simulink model "AnalogOutput_model"  (R2016b)
settings: Solver=FixedStepAuto  StartTime=0.0  StopTime=tFinal  FixedStep=T  RelTol=1e-3  EnableMultiTasking=on
libraries: arduinolib x2
settings Model: SimulationMode=external  ExtModeTrigDuration=100  Creator=Christopher  LastModifiedBy=Christopher
settings DataIOCC: LimitDataPoints=on  StreamToWorkspace=on
settings OptimizationCC: LifeSpan=1  MaxStackSize=64
settings DebuggingCC: AllowSymbolicDim=off  SFUnexpectedBacktrackingDiag=warning  SFNoUnconditionalDefaultTransitionDiag=warning  SFExecutionAtInitializationDiag=none
settings HardwareCC: ProdBitPerPointer=32  ProdBitPerSizeT=32  ProdBitPerPtrDiffT=32  ProdLargestAtomicInteger=Long  ProdLargestAtomicFloat=Double  ProdWordSize=32  ProdHWDeviceType=ARM Compatible->ARM Cortex  UseEmbeddedCoderFeatures=off  UseSimulinkCoderFeatures=off
settings ModelReferenceCC: PropagateSignalLabelsOutOfModel=off
settings RTWCC: SystemTargetFile=ert.tlc  HardwareBoard=Arduino Due  TLCOptions=-aInlineSetEventsForThisBaseRateFcn=TLC_FALSE -aSuppressMultiTaskScheduler=TLC_FALSE -aRateBasedStepFcn=1  TemplateMakefile=ert_default_tmf  Description=Embedded Coder  RTWVerbose=off  Toolchain=Arduino ARM v1.6.7  BuildConfiguration=Faster Runs
settings CodeAppCC: MangleLength=10
settings ERTTargetCC: ERTCustomFileBanners=off  SupportContinuousTime=on  SupportNonInlinedSFcns=on  RemoveResetFunc=off  SupportVariableSizeSignals=on  ModelStepFunctionPrototypeControlCompliant=off  ExtMode=on  ExtModeMexArgs='127.0.0.1' 0 17725  ERTSrcFileBannerTemplate=codertarget_code_template.cgt  ERTHdrFileBannerTemplate=codertarget_code_template.cgt  ERTDataSrcFileTemplate=codertarget_code_template.cgt  ERTDataHdrFileTemplate=codertarget_code_template.cgt  ConvertIfToSwitch=off  SuppressUnreachableDefaultCases=off
settings ConfigComp: CovMetricSettings=dw  CovHtmlReporting=on  CovSaveCumulativeToWorkspaceVar=on  CovSaveSingleToWorkspaceVar=on  CovExternalEMLEnable=off

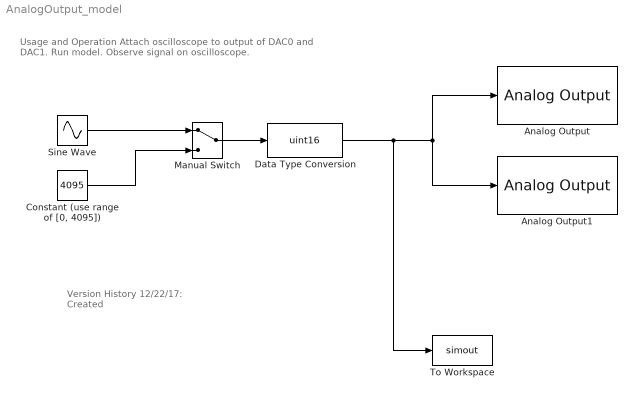
== system AnalogOutput_model ==
  note: Usage and Operation
      | Attach oscilloscope to output of DAC0 and DAC1.
      | Run model.
      | Observe signal on oscilloscope.
  note: Version History
      | 12/22/17: Created
  Analog Output : arduinolib/Analog Output  DACpin=DAC0  blockPlatform=arduino
  Analog Output1 : arduinolib/Analog Output  DACpin=DAC1  blockPlatform=arduino
  "Constant (use range of [0, 4095])" : Constant  Value=4095
  Data Type Conversion : DataTypeConversion  OutDataTypeStr=uint16
  Manual Switch : ManualSwitch
  Sine Wave : Sin  Amplitude=(2^12)/2  Bias=(2^12)/2  Frequency=3  SampleTime=0
  To Workspace : ToWorkspace  VariableName=simout  SaveFormat=Structure With Time  SampleTime=-1
  wires:
  Data Type Conversion/1 -> Analog Output1/1, Analog Output/1, To Workspace/1
  Manual Switch/1 -> Data Type Conversion/1
  Sine Wave/1 -> Manual Switch/1
  "Constant (use range of [0, 4095])"/1 -> Manual Switch/2
